simulink model "modelSys"  (R2016a)
settings: Solver=VariableStepAuto  StartTime=0.0  StopTime=10.0  RelTol=1e-3
values from neighbouring files (symbols this model uses):
  SW = 1    [domaci2.m]
  Tf = 100    [domaci2.m]
settings Model: Creator=milos  LastModifiedBy=milos

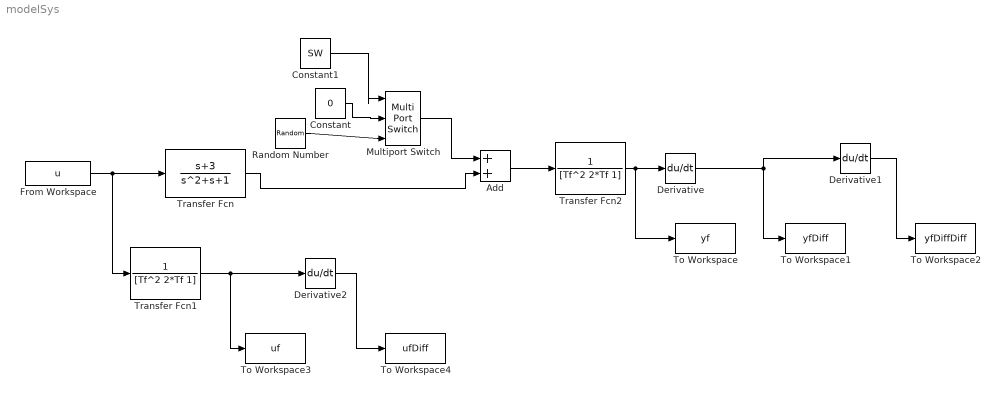
== system modelSys ==
  Add : Sum
  Constant : Constant  Value=0
  Constant1 : Constant  Value=SW
  Derivative : Derivative
  Derivative1 : Derivative
  Derivative2 : Derivative
  From Workspace : FromWorkspace  VariableName=u  SampleTime=0
  Multiport Switch : MultiPortSwitch  Inputs=2
  Random Number : RandomNumber  Variance=0.2
  To Workspace : ToWorkspace  VariableName=yf  SaveFormat=Structure With Time  SampleTime=-1
  To Workspace1 : ToWorkspace  VariableName=yfDiff  SaveFormat=Structure With Time  SampleTime=-1
  To Workspace2 : ToWorkspace  VariableName=yfDiffDiff  SaveFormat=Structure With Time  SampleTime=-1
  To Workspace3 : ToWorkspace  VariableName=uf  SaveFormat=Structure With Time  SampleTime=-1
  To Workspace4 : ToWorkspace  VariableName=ufDiff  SaveFormat=Structure With Time  SampleTime=-1
  Transfer Fcn : TransferFcn  Numerator=[1 3]  Denominator=[1 1 1]
  Transfer Fcn1 : TransferFcn  Denominator=[Tf^2 2*Tf 1]
  Transfer Fcn2 : TransferFcn  Denominator=[Tf^2 2*Tf 1]
  wires:
  Transfer Fcn2/1 -> Derivative/1, To Workspace/1
  Derivative/1 -> Derivative1/1, To Workspace1/1
  Derivative1/1 -> To Workspace2/1
  From Workspace/1 -> Transfer Fcn1/1, Transfer Fcn/1
  Transfer Fcn1/1 -> To Workspace3/1, Derivative2/1
  Derivative2/1 -> To Workspace4/1
  Add/1 -> Transfer Fcn2/1
  Transfer Fcn/1 -> Add/2
  Multiport Switch/1 -> Add/1
  Random Number/1 -> Multiport Switch/3
  Constant/1 -> Multiport Switch/2
  Constant1/1 -> Multiport Switch/1
